simulink model "recursive"  (Simulink 9.1)
settings: Solver=VariableStepDiscrete  StartTime=0.0  StopTime=20.0  RelTol=1e-3  EnableMultiTasking=on
settings Model: Creator=Admin  LastModifiedBy=Asus
settings DataIOCC: LimitDataPoints=on  SignalLoggingSaveFormat=ModelDataLogs
settings OptimizationCC: ExpressionDepthLimit=2147483647  InitFltsAndDblsToZero=on
settings DebuggingCC: SaveWithParameterizedLinksMsg=none  SignalResolutionControl=TryResolveAllWithWarning  SolverPrmCheckMsg=warning  MultiTaskDSMMsg=warning  MultiTaskCondExecSysMsg=none  FcnCallInpInsideContextMsg=warning  StateNameClashWarn=warning
settings GRTTargetCC: TargetFcnLib=ansi_tfl_tmw.mat  GeneratePreprocessorConditionals=Disable all

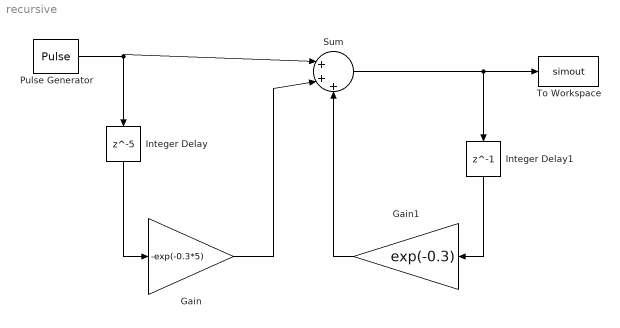
== system recursive ==
  Gain : Gain  Gain=-exp(-0.3*5)
  Gain1 : Gain  Gain=exp(-0.3)
  Integer Delay : Delay  DelayLength=5  InputProcessing=Inherited
  Integer Delay1 : Delay  DelayLength=1  InputProcessing=Inherited
  Pulse Generator : DiscretePulseGenerator  Period=100
  Sum : Sum  Inputs=|+++
  To Workspace : ToWorkspace  VariableName=simout  SampleTime=-1
  wires:
  Integer Delay/1 -> Gain/1
  Gain1/1 -> Sum/3
  Integer Delay1/1 -> Gain1/1
  Sum/1 -> Integer Delay1/1, To Workspace/1
  Pulse Generator/1 -> Integer Delay/1, Sum/1
  Gain/1 -> Sum/2
